simulink model "test_kat_adc_fab_inter"  (Simulink 7.2)
settings: Solver=ode45  StartTime=0.0  StopTime=10.0  RelTol=1e-3
libraries: xbsIndex_r4 x171, simulink x58, dspsigops x24, xps_library x5, casper_library_scopes x2
settings Model: Creator=dave  LastModifiedBy=root
settings OptimizationCC: InitFltsAndDblsToZero=on

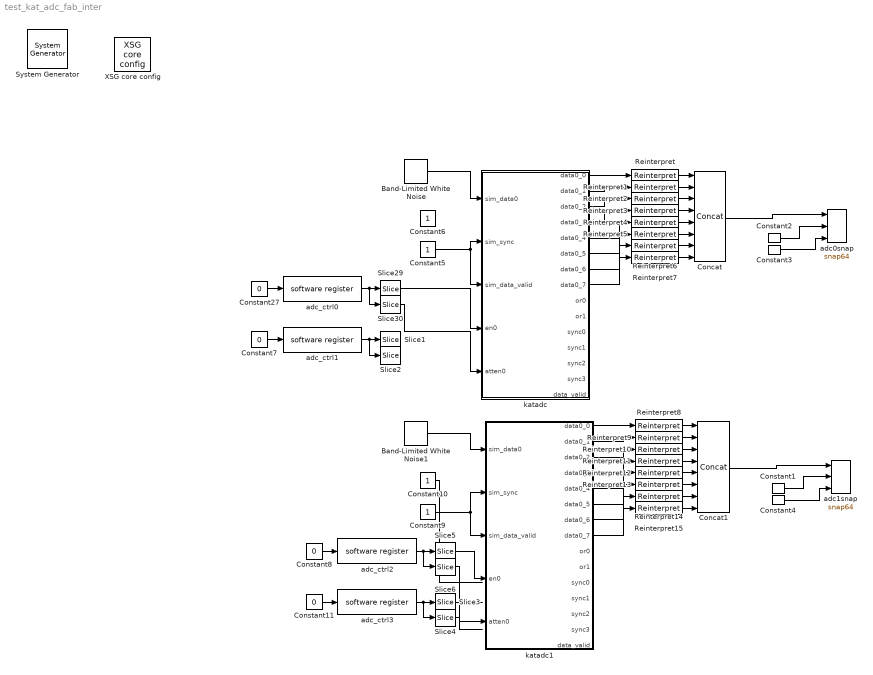
== system test_kat_adc_fab_inter ==
  " System Generator" : xbsIndex_r4/ System Generator  Tag=genX  SystemSampleTime=-1  xilinxfamily=virtex5  part=xc5vsx95t  speed=-1  package=ff1136  synthesis_tool=XST  clock_wrapper=Clock Enables  directory=./test_kat_adc_fab_inter/sysgen  testbench=off  simulink_period=1  sysclk_period=4  dcm_input_clock_period=100  incr_netlist=off  trim_vbits=Everywhere in SubSystem  dbl_ovrd=According to Block Masks  core_generation=According to Block Masks  run_coregen=off  deprecated_control=off  eval_field=0  block_type=sysgen
      settings: block_version=10.1.3
  Band-Limited White Noise : simulink/Sources/Band-Limited White Noise  SystemSampleTime=-1  Cov=[0.1]  Ts=0.25  seed=[23341]
  Band-Limited White Noise1 : simulink/Sources/Band-Limited White Noise  SystemSampleTime=-1  Cov=[0.1]  Ts=0.25  seed=[23341]
  Concat : xbsIndex_r4/Concat  num_inputs=8  dbl_ovrd=off  block_type=concat
      settings: block_version=11.3
  Concat1 : xbsIndex_r4/Concat  num_inputs=8  dbl_ovrd=off  block_type=concat
      settings: block_version=11.3
  Constant{1..4} (4 alike) : xbsIndex_r4/Constant  arith_type=Boolean  const=0  n_bits=16  bin_pt=14  explicit_period=on  period=1  equ=P=C  opselect=C  inp2=PCIN>>17  opr=+  inp1=P  carry=CIN  dbl_ovrd=off  block_type=constant
      settings: block_version=11.3
  Constant{5..6,9..10} (4 alike) : Constant  OutDataType=sfix(16)  OutScaling=2^0  SampleTime=1
  Constant{7..8,11,27} (4 alike) : Constant  Value=0  OutDataType=sfix(16)  OutScaling=2^0
  Reinterpret{,1..15} (16 alike) : xbsIndex_r4/Reinterpret  force_arith_type=on  arith_type=Unsigned  force_bin_pt=on  bin_pt=0  block_type=reinterpret
      settings: infoedit="Changes signal type without altering the binary representation.   You can changed the signal between signed and unsigned, and relocate the binary point.<br><br>Hardware notes: In hardware this block costs nothing.<br><br>Example:  Suppose the input is 6 bits wide, signed, with 2 fractional bits, and the output is forced to unsigned with 0 fractional bits.  Then an input of -2.0 (1110.00 in binary 2's complement) becomes an output of 56 (111000 in binary)."  block_version=11.3
  Slice{1,3,5,29} (4 alike) : xbsIndex_r4/Slice  nbits=1  boolean_output=on  mode=Upper Bit Location + Width  bit1=0  base1=MSB of Input  bit0=0  base0=LSB of Input  dbl_ovrd=off  block_type=slice
  Slice{2,4,6,30} (4 alike) : xbsIndex_r4/Slice  nbits=6  boolean_output=off  mode=Lower Bit Location + Width  bit1=0  base1=MSB of Input  bit0=0  base0=LSB of Input  dbl_ovrd=off  block_type=slice
  XSG core config : xps_library/XSG core config  Tag=xps:xsg  SystemSampleTime=-1  hw_sys=ROACH:sx95t  ibob_linux=off  clk_src=adc0_clk  iBOB_clk_src=sys_clk  BEE2_ctrl_clk_src=sys_clk  BEE2_usr_clk_src=sys_clk  ROACH_clk_src=adc0_clk  CORR_clk_src=sys_clk  gpio_clk_io_group=iBOB:sma  gpio_clk_bit_index=0  clk_rate=250  sample_period=1  synthesis_tool=XST  mpc_type=powerpc440_ext
  adc0snap : casper_library_scopes/snap64  SystemSampleTime=-1  nsamples=11
  adc1snap : casper_library_scopes/snap64  SystemSampleTime=-1  nsamples=11
  adc_ctrl0 : xps_library/software register  Tag=xps:sw_reg  SystemSampleTime=-1  io_dir=From Processor  arith_type=Unsigned  bitwidth=32  bin_pt=0  sample_period=1  gw_name=test_kat_adc_fab_inter_adc_ctrl0_user_data_out
      link override poco_cd_tr0_ld_time_msb_user_data_out: arith_type=Unsigned  n_bits=32  bin_pt=0  period=1
      link override poco_dram_vacc_r001_cd_tr0_ld_time_msb_user_data_out: arith_type=Unsigned  n_bits=32  bin_pt=0  period=1
      link override poco_dram_vacc_r002_cd_tr0_ld_time_msb_user_data_out: arith_type=Unsigned  n_bits=32  bin_pt=0  period=1
      link override poco_dram_vacc_r003_cd_tr0_ld_time_msb_user_data_out: arith_type=Unsigned  n_bits=32  bin_pt=0  period=1
      link override poco_dram_vacc_r004_cd_tr0_ld_time_msb_user_data_out: arith_type=Unsigned  n_bits=32  bin_pt=0  period=1
      link override poco_dram_vacc_r005_cd_tr0_ld_time_msb_user_data_out: arith_type=Unsigned  n_bits=32  bin_pt=0  period=1
      link override poco_dram_vacc_r006_cd_tr0_ld_time_msb_user_data_out: arith_type=Unsigned  n_bits=32  bin_pt=0  period=1
      link override poco_r006_cd_tr0_ld_time_msb_user_data_out: arith_type=Unsigned  n_bits=32  bin_pt=0  period=1
      link override poco_red_cd_ld_time_msb_user_data_out: arith_type=Unsigned  n_bits=32  bin_pt=0  period=1
      link override poco_ref_roach_adc0_cd_ld_time_msb_user_data_out: arith_type=Unsigned  n_bits=32  bin_pt=0  period=1
      link override poco_ref_roach_reduced_adc0_cd_ld_time_msb_user_data_out: arith_type=Unsigned  n_bits=32  bin_pt=0  period=1
      link override poco_roach_cd_tr0_ld_time_msb_user_data_out: arith_type=Unsigned  n_bits=32  bin_pt=0  period=1
      link override poco_roach_r006_cd_tr0_ld_time_msb_user_data_out: arith_type=Unsigned  n_bits=32  bin_pt=0  period=1
      link override poco_roach_r007_cd_tr0_ld_time_msb_user_data_out: arith_type=Unsigned  n_bits=32  bin_pt=0  period=1
      link override poco_roach_red_adc0_cd_ld_time_msb_user_data_out: arith_type=Unsigned  n_bits=32  bin_pt=0  period=1
      link override poco_roach_vacc_r006_cd_tr0_ld_time_msb_user_data_out: arith_type=Unsigned  n_bits=32  bin_pt=0  period=1
  adc_ctrl1 : xps_library/software register  Tag=xps:sw_reg  SystemSampleTime=-1  io_dir=From Processor  arith_type=Unsigned  bitwidth=32  bin_pt=0  sample_period=1  gw_name=test_kat_adc_fab_inter_adc_ctrl1_user_data_out
      link override poco_cd_tr0_ld_time_msb_user_data_out: arith_type=Unsigned  n_bits=32  bin_pt=0  period=1
      link override poco_dram_vacc_r001_cd_tr0_ld_time_msb_user_data_out: arith_type=Unsigned  n_bits=32  bin_pt=0  period=1
      link override poco_dram_vacc_r002_cd_tr0_ld_time_msb_user_data_out: arith_type=Unsigned  n_bits=32  bin_pt=0  period=1
      link override poco_dram_vacc_r003_cd_tr0_ld_time_msb_user_data_out: arith_type=Unsigned  n_bits=32  bin_pt=0  period=1
      link override poco_dram_vacc_r004_cd_tr0_ld_time_msb_user_data_out: arith_type=Unsigned  n_bits=32  bin_pt=0  period=1
      link override poco_dram_vacc_r005_cd_tr0_ld_time_msb_user_data_out: arith_type=Unsigned  n_bits=32  bin_pt=0  period=1
      link override poco_dram_vacc_r006_cd_tr0_ld_time_msb_user_data_out: arith_type=Unsigned  n_bits=32  bin_pt=0  period=1
      link override poco_r006_cd_tr0_ld_time_msb_user_data_out: arith_type=Unsigned  n_bits=32  bin_pt=0  period=1
      link override poco_red_cd_ld_time_msb_user_data_out: arith_type=Unsigned  n_bits=32  bin_pt=0  period=1
      link override poco_ref_roach_adc0_cd_ld_time_msb_user_data_out: arith_type=Unsigned  n_bits=32  bin_pt=0  period=1
      link override poco_ref_roach_reduced_adc0_cd_ld_time_msb_user_data_out: arith_type=Unsigned  n_bits=32  bin_pt=0  period=1
      link override poco_roach_cd_tr0_ld_time_msb_user_data_out: arith_type=Unsigned  n_bits=32  bin_pt=0  period=1
      link override poco_roach_r006_cd_tr0_ld_time_msb_user_data_out: arith_type=Unsigned  n_bits=32  bin_pt=0  period=1
      link override poco_roach_r007_cd_tr0_ld_time_msb_user_data_out: arith_type=Unsigned  n_bits=32  bin_pt=0  period=1
      link override poco_roach_red_adc0_cd_ld_time_msb_user_data_out: arith_type=Unsigned  n_bits=32  bin_pt=0  period=1
      link override poco_roach_vacc_r006_cd_tr0_ld_time_msb_user_data_out: arith_type=Unsigned  n_bits=32  bin_pt=0  period=1
  adc_ctrl2 : xps_library/software register  Tag=xps:sw_reg  SystemSampleTime=-1  io_dir=From Processor  arith_type=Unsigned  bitwidth=32  bin_pt=0  sample_period=1  gw_name=test_kat_adc_fab_inter_adc_ctrl2_user_data_out
      link override poco_cd_tr0_ld_time_msb_user_data_out: arith_type=Unsigned  n_bits=32  bin_pt=0  period=1
      link override poco_dram_vacc_r001_cd_tr0_ld_time_msb_user_data_out: arith_type=Unsigned  n_bits=32  bin_pt=0  period=1
      link override poco_dram_vacc_r002_cd_tr0_ld_time_msb_user_data_out: arith_type=Unsigned  n_bits=32  bin_pt=0  period=1
      link override poco_dram_vacc_r003_cd_tr0_ld_time_msb_user_data_out: arith_type=Unsigned  n_bits=32  bin_pt=0  period=1
      link override poco_dram_vacc_r004_cd_tr0_ld_time_msb_user_data_out: arith_type=Unsigned  n_bits=32  bin_pt=0  period=1
      link override poco_dram_vacc_r005_cd_tr0_ld_time_msb_user_data_out: arith_type=Unsigned  n_bits=32  bin_pt=0  period=1
      link override poco_dram_vacc_r006_cd_tr0_ld_time_msb_user_data_out: arith_type=Unsigned  n_bits=32  bin_pt=0  period=1
      link override poco_r006_cd_tr0_ld_time_msb_user_data_out: arith_type=Unsigned  n_bits=32  bin_pt=0  period=1
      link override poco_red_cd_ld_time_msb_user_data_out: arith_type=Unsigned  n_bits=32  bin_pt=0  period=1
      link override poco_ref_roach_adc0_cd_ld_time_msb_user_data_out: arith_type=Unsigned  n_bits=32  bin_pt=0  period=1
      link override poco_ref_roach_reduced_adc0_cd_ld_time_msb_user_data_out: arith_type=Unsigned  n_bits=32  bin_pt=0  period=1
      link override poco_roach_cd_tr0_ld_time_msb_user_data_out: arith_type=Unsigned  n_bits=32  bin_pt=0  period=1
      link override poco_roach_r006_cd_tr0_ld_time_msb_user_data_out: arith_type=Unsigned  n_bits=32  bin_pt=0  period=1
      link override poco_roach_r007_cd_tr0_ld_time_msb_user_data_out: arith_type=Unsigned  n_bits=32  bin_pt=0  period=1
      link override poco_roach_red_adc0_cd_ld_time_msb_user_data_out: arith_type=Unsigned  n_bits=32  bin_pt=0  period=1
      link override poco_roach_vacc_r006_cd_tr0_ld_time_msb_user_data_out: arith_type=Unsigned  n_bits=32  bin_pt=0  period=1
  adc_ctrl3 : xps_library/software register  Tag=xps:sw_reg  SystemSampleTime=-1  io_dir=From Processor  arith_type=Unsigned  bitwidth=32  bin_pt=0  sample_period=1  gw_name=test_kat_adc_fab_inter_adc_ctrl3_user_data_out
      link override poco_cd_tr0_ld_time_msb_user_data_out: arith_type=Unsigned  n_bits=32  bin_pt=0  period=1
      link override poco_dram_vacc_r001_cd_tr0_ld_time_msb_user_data_out: arith_type=Unsigned  n_bits=32  bin_pt=0  period=1
      link override poco_dram_vacc_r002_cd_tr0_ld_time_msb_user_data_out: arith_type=Unsigned  n_bits=32  bin_pt=0  period=1
      link override poco_dram_vacc_r003_cd_tr0_ld_time_msb_user_data_out: arith_type=Unsigned  n_bits=32  bin_pt=0  period=1
      link override poco_dram_vacc_r004_cd_tr0_ld_time_msb_user_data_out: arith_type=Unsigned  n_bits=32  bin_pt=0  period=1
      link override poco_dram_vacc_r005_cd_tr0_ld_time_msb_user_data_out: arith_type=Unsigned  n_bits=32  bin_pt=0  period=1
      link override poco_dram_vacc_r006_cd_tr0_ld_time_msb_user_data_out: arith_type=Unsigned  n_bits=32  bin_pt=0  period=1
      link override poco_r006_cd_tr0_ld_time_msb_user_data_out: arith_type=Unsigned  n_bits=32  bin_pt=0  period=1
      link override poco_red_cd_ld_time_msb_user_data_out: arith_type=Unsigned  n_bits=32  bin_pt=0  period=1
      link override poco_ref_roach_adc0_cd_ld_time_msb_user_data_out: arith_type=Unsigned  n_bits=32  bin_pt=0  period=1
      link override poco_ref_roach_reduced_adc0_cd_ld_time_msb_user_data_out: arith_type=Unsigned  n_bits=32  bin_pt=0  period=1
      link override poco_roach_cd_tr0_ld_time_msb_user_data_out: arith_type=Unsigned  n_bits=32  bin_pt=0  period=1
      link override poco_roach_r006_cd_tr0_ld_time_msb_user_data_out: arith_type=Unsigned  n_bits=32  bin_pt=0  period=1
      link override poco_roach_r007_cd_tr0_ld_time_msb_user_data_out: arith_type=Unsigned  n_bits=32  bin_pt=0  period=1
      link override poco_roach_red_adc0_cd_ld_time_msb_user_data_out: arith_type=Unsigned  n_bits=32  bin_pt=0  period=1
      link override poco_roach_vacc_r006_cd_tr0_ld_time_msb_user_data_out: arith_type=Unsigned  n_bits=32  bin_pt=0  period=1
  katadc : Subsystem  Tag=xps:katadc  AncestorBlock=xps_library/katadc  mask(katadc){adc_brd=adc0, adc_interleave=on, bypass_auto=off, en_gain=on, adc_clk_rate=900, sample_period=1}
      mask prompts: adc_brd "ADC board"; adc_interleave "ADC interleave mode"; bypass_auto "Bypass auto config"; en_gain "Enable gain"; adc_clk_rate "ADC sampling rate (MHz)"; sample_period "Sample period"
      mask init:
      | name = gcb;
      | katadc_init(gcb, ...
      |     'name', name, ...
      |     'adc_brd', adc_brd, ...
      |     'adc_interleave', adc_interleave, ...
      |     'bypass_auto', bypass_auto, ...
      |     'en_gain', en_gain, ...
      |     'adc_clk_rate', adc_clk_rate, ...
      |     'sample_period', sample_period);
      mask StyleString: popup(adc0|adc1),checkbox,checkbox,checkbox,edit,edit
  katadc1 : Subsystem  Tag=xps:katadc  AncestorBlock=xps_library/katadc  mask(katadc){adc_brd=adc1, adc_interleave=on, bypass_auto=on, en_gain=on, adc_clk_rate=900, sample_period=1}
      mask prompts: adc_brd "ADC board"; adc_interleave "ADC interleave mode"; bypass_auto "Bypass auto config"; en_gain "Enable gain"; adc_clk_rate "ADC sampling rate (MHz)"; sample_period "Sample period"
      mask init: same as test_kat_adc_fab_inter/katadc
      mask StyleString: popup(adc0|adc1),checkbox,checkbox,checkbox,edit,edit
  wires:
  Reinterpret/1 -> Concat/1
  Reinterpret1/1 -> Concat/2
  Reinterpret2/1 -> Concat/3
  Reinterpret3/1 -> Concat/4
  Reinterpret4/1 -> Concat/5
  Reinterpret5/1 -> Concat/6
  Reinterpret6/1 -> Concat/7
  Reinterpret7/1 -> Concat/8
  Concat/1 -> adc0snap/1
  Constant2/1 -> adc0snap/2
  Constant3/1 -> adc0snap/3
  Reinterpret8/1 -> Concat1/1
  Reinterpret9/1 -> Concat1/2
  Reinterpret10/1 -> Concat1/3
  Reinterpret11/1 -> Concat1/4
  Reinterpret12/1 -> Concat1/5
  Reinterpret13/1 -> Concat1/6
  Reinterpret14/1 -> Concat1/7
  Reinterpret15/1 -> Concat1/8
  Concat1/1 -> adc1snap/1
  Constant1/1 -> adc1snap/2
  Constant4/1 -> adc1snap/3
  Constant5/1 -> katadc/2(sim_sync), katadc/3(sim_data_valid)
  Band-Limited White Noise/1 -> katadc/1(sim_data0)
  Constant27/1 -> adc_ctrl0/1
  adc_ctrl0/1 -> Slice29/1, Slice30/1
  Slice29/1 -> katadc/4(en0)
  Slice30/1 -> katadc/5(atten0)
  Constant7/1 -> adc_ctrl1/1
  adc_ctrl1/1 -> Slice2/1, Slice1/1
  Constant9/1 -> katadc1/2(sim_sync), katadc1/3(sim_data_valid)
  Constant10/1 -> ?
  Band-Limited White Noise1/1 -> katadc1/1(sim_data0)
  Constant8/1 -> adc_ctrl2/1
  adc_ctrl2/1 -> Slice5/1, Slice6/1
  Slice5/1 -> katadc1/4(en0)
  Slice6/1 -> katadc1/5(atten0)
  Constant11/1 -> adc_ctrl3/1
  adc_ctrl3/1 -> Slice4/1, Slice3/1
  Slice3/1 -> ?
  Slice4/1 -> ?
  katadc/1(data0_0) -> Reinterpret/1
  katadc/2(data0_1) -> Reinterpret1/1
  katadc/3(data0_2) -> Reinterpret2/1
  katadc/4(data0_3) -> Reinterpret3/1
  katadc/5(data0_4) -> Reinterpret4/1
  katadc/6(data0_5) -> Reinterpret5/1
  katadc/7(data0_6) -> Reinterpret6/1
  katadc/8(data0_7) -> Reinterpret7/1
  katadc1/1(data0_0) -> Reinterpret8/1
  katadc1/2(data0_1) -> Reinterpret9/1
  katadc1/3(data0_2) -> Reinterpret10/1
  katadc1/4(data0_3) -> Reinterpret11/1
  katadc1/5(data0_4) -> Reinterpret12/1
  katadc1/6(data0_5) -> Reinterpret13/1
  katadc1/7(data0_6) -> Reinterpret14/1
  katadc1/8(data0_7) -> Reinterpret15/1

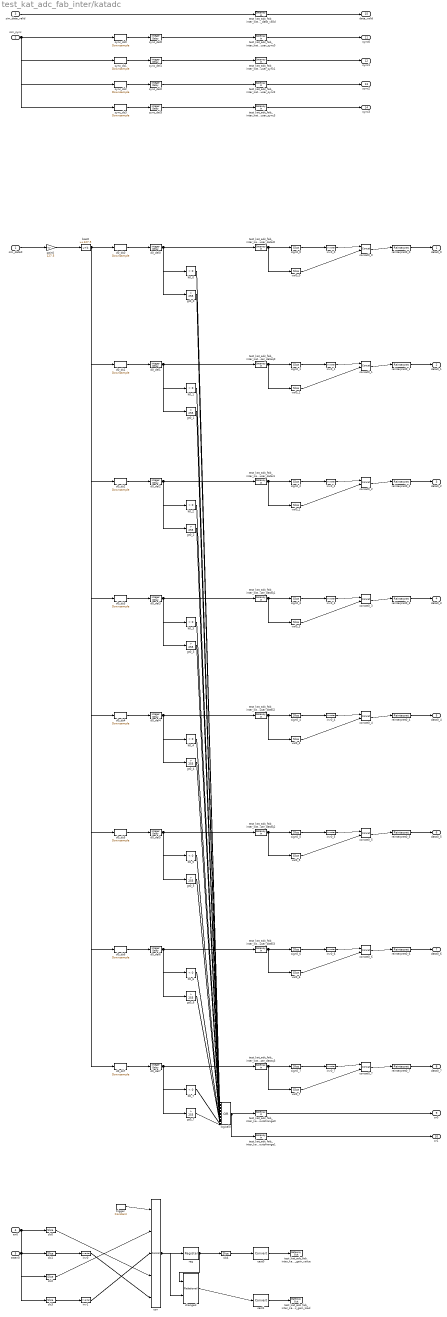
== system test_kat_adc_fab_inter/katadc ==
  sim_data0 : Inport
  sim_sync : Inport  Port=2
  sim_data_valid : Inport  Port=3
  en0 : Inport  Port=4
  atten0 : Inport  Port=5
  bias0 : Bias  Bias=127.5  SaturateOnIntegerOverflow=on
  cast0 : xbsIndex_r4/Convert  arith_type=Unsigned  n_bits=14  bin_pt=0  quantization=Truncate  overflow=Wrap  latency=0  dbl_ovrd=off  pipeline=off  block_type=convert
      settings: block_version=11.4
  cast1 : xbsIndex_r4/Convert  arith_type=Boolean  n_bits=16  bin_pt=14  quantization=Truncate  overflow=Wrap  latency=0  dbl_ovrd=off  pipeline=off  block_type=convert
      settings: block_version=11.4
  changed : xbsIndex_r4/Relational  mode=a!=b  en=off  latency=1  dbl_ovrd=off  block_type=relational
  con : xbsIndex_r4/Concat  num_inputs=5  dbl_ovrd=off  block_type=concat
  concat0_{0..7} (8 alike) : xbsIndex_r4/Concat  num_inputs=2  dbl_ovrd=off  block_type=concat
  d0_del0 : simulink/Discrete/Integer Delay  vinit=0.0  samptime=-1  NumDelays=2
  d0_del{1..7} (7 alike) : simulink/Discrete/Integer Delay  vinit=0.0  samptime=-1  NumDelays=1
  d0_ds0 : dspsigops/Downsample  N=8  phase=0  ic=0  smode=Allow multirate  fmode=Maintain input frame size
  d0_ds1 : dspsigops/Downsample  N=8  phase=1  ic=0  smode=Allow multirate  fmode=Maintain input frame size
  d0_ds2 : dspsigops/Downsample  N=8  phase=2  ic=0  smode=Allow multirate  fmode=Maintain input frame size
  d0_ds3 : dspsigops/Downsample  N=8  phase=3  ic=0  smode=Allow multirate  fmode=Maintain input frame size
  d0_ds4 : dspsigops/Downsample  N=8  phase=4  ic=0  smode=Allow multirate  fmode=Maintain input frame size
  d0_ds5 : dspsigops/Downsample  N=8  phase=5  ic=0  smode=Allow multirate  fmode=Maintain input frame size
  d0_ds6 : dspsigops/Downsample  N=8  phase=6  ic=0  smode=Allow multirate  fmode=Maintain input frame size
  d0_ds7 : dspsigops/Downsample  N=8  phase=7  ic=0  smode=Allow multirate  fmode=Maintain input frame size
  gain0 : Gain  Gain=127.5  SaturateOnIntegerOverflow=on  OutDataTypeStr=Inherit: Same as input  ParamDataTypeStr=Inherit: Same as input
  gt0_{0..7} (8 alike) : simulink/Logic and Bit Operations/Compare To Constant  SystemSampleTime=-1  relop=>  const=255  LogicOutDataTypeMode=boolean  ZeroCross=off
  inv0 : xbsIndex_r4/Inverter  en=off  latency=0  dbl_ovrd=off  block_type=inv
      settings: block_version=11.4
  inv0_{0..7} (8 alike) : xbsIndex_r4/Inverter  en=off  latency=0  dbl_ovrd=off  block_type=inv
      settings: block_version=11.4
  inv1 : xbsIndex_r4/Inverter  en=off  latency=0  dbl_ovrd=off  block_type=inv
      settings: block_version=11.4
  logical0 : Logic  Operator=OR  Inputs=16  AllPortsSameDT=off  OutDataTypeMode=boolean  OutDataTypeStr=boolean
  lt0_{0..7} (8 alike) : simulink/Logic and Bit Operations/Compare To Constant  SystemSampleTime=-1  relop=<  const=0  LogicOutDataTypeMode=boolean  ZeroCross=off
  reg : xbsIndex_r4/Register  init=0  rst=off  en=off  dbl_ovrd=off  block_type=register
      settings: block_version=11.4
  reinterpret0_{0..7} (8 alike) : xbsIndex_r4/Reinterpret  force_arith_type=on  arith_type="Signed  (2's comp)"  force_bin_pt=on  bin_pt=7  block_type=reinterpret
      settings: infoedit="Changes signal type without altering the binary representation.   You can changed the signal between signed and unsigned, and relocate the binary point.<br><br>Hardware notes: In hardware this block costs nothing.<br><br>Example:  Suppose the input is 6 bits wide, signed, with 2 fractional bits, and the output is forced to unsigned with 0 fractional bits.  Then an input of -2.0 (1110.00 in binary 2's complement) becomes an output of 56 (111000 in binary)."
  sign0_{0..7} (8 alike) : xbsIndex_r4/Slice  nbits=1  boolean_output=off  mode=Upper Bit Location + Width  bit1=0  base1=MSB of Input  bit0=0  base0=MSB of Input  dbl_ovrd=off  block_type=slice
  slc0 : xbsIndex_r4/Slice  nbits=1  boolean_output=off  mode=Lower Bit Location + Width  bit1=0  base1=MSB of Input  bit0=0  base0=LSB of Input  dbl_ovrd=off  block_type=slice
  slc1 : xbsIndex_r4/Slice  nbits=6  boolean_output=off  mode=Lower Bit Location + Width  bit1=0  base1=MSB of Input  bit0=0  base0=LSB of Input  dbl_ovrd=off  block_type=slice
  slc2 : xbsIndex_r4/Slice  nbits=1  boolean_output=off  mode=Lower Bit Location + Width  bit1=0  base1=MSB of Input  bit0=0  base0=LSB of Input  dbl_ovrd=off  block_type=slice
  slc3 : xbsIndex_r4/Slice  nbits=6  boolean_output=off  mode=Lower Bit Location + Width  bit1=0  base1=MSB of Input  bit0=0  base0=LSB of Input  dbl_ovrd=off  block_type=slice
  slc4 : xbsIndex_r4/Slice  nbits=14  boolean_output=off  mode=Lower Bit Location + Width  bit1=0  base1=MSB of Input  bit0=0  base0=LSB of Input  dbl_ovrd=off  block_type=slice
  sync_del0 : simulink/Discrete/Integer Delay  vinit=0.0  samptime=-1  NumDelays=2
  sync_del1 : simulink/Discrete/Integer Delay  vinit=0.0  samptime=-1  NumDelays=1
  sync_del2 : simulink/Discrete/Integer Delay  vinit=0.0  samptime=-1  NumDelays=1
  sync_del3 : simulink/Discrete/Integer Delay  vinit=0.0  samptime=-1  NumDelays=1
  sync_ds0 : dspsigops/Downsample  N=8  phase=0  ic=0  smode=Allow multirate  fmode=Maintain input frame size
  sync_ds1 : dspsigops/Downsample  N=8  phase=2  ic=0  smode=Allow multirate  fmode=Maintain input frame size
  sync_ds2 : dspsigops/Downsample  N=8  phase=4  ic=0  smode=Allow multirate  fmode=Maintain input frame size
  sync_ds3 : dspsigops/Downsample  N=8  phase=6  ic=0  smode=Allow multirate  fmode=Maintain input frame size
  test_kat_adc_fab_inter_katadc_gain_load : xbsIndex_r4/Gateway Out  hdl_port=on  timing_constraint=None  locs_specified=off  LOCs={}  block_type=gatewayout
      settings: infoedit="Gateway out block.  Converts Xilinx fixed point inputs into ouputs of type Simulink integer, double, or fixed point.<br><br>Hardware notes:  In hardware these blocks become top level output ports or are discarded, depending on how they are configured."  block_version=11.4
  test_kat_adc_fab_inter_katadc_gain_value : xbsIndex_r4/Gateway Out  hdl_port=on  timing_constraint=None  locs_specified=off  LOCs={}  block_type=gatewayout
      settings: infoedit="Gateway out block.  Converts Xilinx fixed point inputs into ouputs of type Simulink integer, double, or fixed point.<br><br>Hardware notes:  In hardware these blocks become top level output ports or are discarded, depending on how they are configured."  block_version=11.4
  test_kat_adc_fab_inter_katadc_user_data_valid : xbsIndex_r4/Gateway In  arith_type=Boolean  n_bits=16  bin_pt=14  quantization="Round  (unbiased: +/- Inf)"  overflow=Saturate  period=1  dbl_ovrd=off  timing_constraint=None  locs_specified=off  LOCs={}  hdl_port=on  block_type=gatewayin
      settings: infoedit="Gateway in block.  Converts inputs of type Simulink integer, double and fixed point to  Xilinx fixed point type.<br><br>Hardware notes:  In hardware these blocks become top level input ports."  block_version=11.4
  test_kat_adc_fab_inter_katadc_user_datai{0..3} (4 alike) : xbsIndex_r4/Gateway In  arith_type="Signed  (2's comp)"  n_bits=8  bin_pt=0  quantization="Round  (unbiased: +/- Inf)"  overflow=Saturate  period=1  dbl_ovrd=off  timing_constraint=None  locs_specified=off  LOCs={}  hdl_port=on  block_type=gatewayin
      settings: infoedit="Gateway in block.  Converts inputs of type Simulink integer, double and fixed point to  Xilinx fixed point type.<br><br>Hardware notes:  In hardware these blocks become top level input ports."  block_version=11.4
  test_kat_adc_fab_inter_katadc_user_dataq{0..3} (4 alike) : xbsIndex_r4/Gateway In  arith_type="Signed  (2's comp)"  n_bits=8  bin_pt=0  quantization="Round  (unbiased: +/- Inf)"  overflow=Saturate  period=1  dbl_ovrd=off  timing_constraint=None  locs_specified=off  LOCs={}  hdl_port=on  block_type=gatewayin
      settings: infoedit="Gateway in block.  Converts inputs of type Simulink integer, double and fixed point to  Xilinx fixed point type.<br><br>Hardware notes:  In hardware these blocks become top level input ports."  block_version=11.4
  test_kat_adc_fab_inter_katadc_user_outofrange0 : xbsIndex_r4/Gateway In  arith_type=Boolean  n_bits=16  bin_pt=14  quantization="Round  (unbiased: +/- Inf)"  overflow=Saturate  period=1  dbl_ovrd=off  timing_constraint=None  locs_specified=off  LOCs={}  hdl_port=on  block_type=gatewayin
      settings: infoedit="Gateway in block.  Converts inputs of type Simulink integer, double and fixed point to  Xilinx fixed point type.<br><br>Hardware notes:  In hardware these blocks become top level input ports."  block_version=11.4
  test_kat_adc_fab_inter_katadc_user_outofrange1 : xbsIndex_r4/Gateway In  arith_type=Boolean  n_bits=16  bin_pt=14  quantization="Round  (unbiased: +/- Inf)"  overflow=Saturate  period=1  dbl_ovrd=off  timing_constraint=None  locs_specified=off  LOCs={}  hdl_port=on  block_type=gatewayin
      settings: infoedit="Gateway in block.  Converts inputs of type Simulink integer, double and fixed point to  Xilinx fixed point type.<br><br>Hardware notes:  In hardware these blocks become top level input ports."  block_version=11.4
  test_kat_adc_fab_inter_katadc_user_sync{0..3} (4 alike) : xbsIndex_r4/Gateway In  arith_type=Boolean  n_bits=16  bin_pt=14  quantization="Round  (unbiased: +/- Inf)"  overflow=Saturate  period=1  dbl_ovrd=off  timing_constraint=None  locs_specified=off  LOCs={}  hdl_port=on  block_type=gatewayin
      settings: infoedit="Gateway in block.  Converts inputs of type Simulink integer, double and fixed point to  Xilinx fixed point type.<br><br>Hardware notes:  In hardware these blocks become top level input ports."  block_version=11.4
  trigger : xbsIndex_r4/Constant  arith_type=Unsigned  const=1  n_bits=1  bin_pt=0  explicit_period=off  period=1  equ=P=C  opselect=C  inp2=PCIN>>17  opr=+  inp1=P  carry=CIN  dbl_ovrd=off  block_type=constant
      settings: block_version=11.4
  val0_{0..7} (8 alike) : xbsIndex_r4/Slice  nbits=7  boolean_output=off  mode=Lower Bit Location + Width  bit1=0  base1=LSB of Input  bit0=0  base0=LSB of Input  dbl_ovrd=off  block_type=slice
  data0_0 : Outport
  data0_1 : Outport  Port=2
  data0_2 : Outport  Port=3
  data0_3 : Outport  Port=4
  data0_4 : Outport  Port=5
  data0_5 : Outport  Port=6
  data0_6 : Outport  Port=7
  data0_7 : Outport  Port=8
  or0 : Outport  Port=9
  or1 : Outport  Port=10
  sync0 : Outport  Port=11
  sync1 : Outport  Port=12
  sync2 : Outport  Port=13
  sync3 : Outport  Port=14
  data_valid : Outport  Port=15
  wires:
  sim_data0/1 -> gain0/1
  gain0/1 -> bias0/1
  bias0/1 -> d0_ds0/1, d0_ds1/1, d0_ds2/1, d0_ds3/1, d0_ds4/1, d0_ds5/1, d0_ds6/1, d0_ds7/1
  d0_ds0/1 -> d0_del0/1
  d0_del0/1 -> test_kat_adc_fab_inter_katadc_user_datai0/1, lt0_0/1, gt0_0/1
  test_kat_adc_fab_inter_katadc_user_datai0/1 -> sign0_0/1, val0_0/1
  sign0_0/1 -> inv0_0/1
  inv0_0/1 -> concat0_0/1
  val0_0/1 -> concat0_0/2
  concat0_0/1 -> reinterpret0_0/1
  reinterpret0_0/1 -> data0_0/1
  d0_ds1/1 -> d0_del1/1
  d0_del1/1 -> test_kat_adc_fab_inter_katadc_user_dataq0/1, lt0_1/1, gt0_1/1
  test_kat_adc_fab_inter_katadc_user_dataq0/1 -> sign0_1/1, val0_1/1
  sign0_1/1 -> inv0_1/1
  inv0_1/1 -> concat0_1/1
  val0_1/1 -> concat0_1/2
  concat0_1/1 -> reinterpret0_1/1
  reinterpret0_1/1 -> data0_1/1
  d0_ds2/1 -> d0_del2/1
  d0_del2/1 -> test_kat_adc_fab_inter_katadc_user_datai1/1, lt0_2/1, gt0_2/1
  test_kat_adc_fab_inter_katadc_user_datai1/1 -> sign0_2/1, val0_2/1
  sign0_2/1 -> inv0_2/1
  inv0_2/1 -> concat0_2/1
  val0_2/1 -> concat0_2/2
  concat0_2/1 -> reinterpret0_2/1
  reinterpret0_2/1 -> data0_2/1
  d0_ds3/1 -> d0_del3/1
  d0_del3/1 -> test_kat_adc_fab_inter_katadc_user_dataq1/1, lt0_3/1, gt0_3/1
  test_kat_adc_fab_inter_katadc_user_dataq1/1 -> sign0_3/1, val0_3/1
  sign0_3/1 -> inv0_3/1
  inv0_3/1 -> concat0_3/1
  val0_3/1 -> concat0_3/2
  concat0_3/1 -> reinterpret0_3/1
  reinterpret0_3/1 -> data0_3/1
  d0_ds4/1 -> d0_del4/1
  d0_del4/1 -> test_kat_adc_fab_inter_katadc_user_datai2/1, lt0_4/1, gt0_4/1
  test_kat_adc_fab_inter_katadc_user_datai2/1 -> sign0_4/1, val0_4/1
  sign0_4/1 -> inv0_4/1
  inv0_4/1 -> concat0_4/1
  val0_4/1 -> concat0_4/2
  concat0_4/1 -> reinterpret0_4/1
  reinterpret0_4/1 -> data0_4/1
  d0_ds5/1 -> d0_del5/1
  d0_del5/1 -> test_kat_adc_fab_inter_katadc_user_dataq2/1, lt0_5/1, gt0_5/1
  test_kat_adc_fab_inter_katadc_user_dataq2/1 -> sign0_5/1, val0_5/1
  sign0_5/1 -> inv0_5/1
  inv0_5/1 -> concat0_5/1
  val0_5/1 -> concat0_5/2
  concat0_5/1 -> reinterpret0_5/1
  reinterpret0_5/1 -> data0_5/1
  d0_ds6/1 -> d0_del6/1
  d0_del6/1 -> test_kat_adc_fab_inter_katadc_user_datai3/1, lt0_6/1, gt0_6/1
  test_kat_adc_fab_inter_katadc_user_datai3/1 -> sign0_6/1, val0_6/1
  sign0_6/1 -> inv0_6/1
  inv0_6/1 -> concat0_6/1
  val0_6/1 -> concat0_6/2
  concat0_6/1 -> reinterpret0_6/1
  reinterpret0_6/1 -> data0_6/1
  d0_ds7/1 -> d0_del7/1
  d0_del7/1 -> test_kat_adc_fab_inter_katadc_user_dataq3/1, lt0_7/1, gt0_7/1
  test_kat_adc_fab_inter_katadc_user_dataq3/1 -> sign0_7/1, val0_7/1
  sign0_7/1 -> inv0_7/1
  inv0_7/1 -> concat0_7/1
  val0_7/1 -> concat0_7/2
  concat0_7/1 -> reinterpret0_7/1
  reinterpret0_7/1 -> data0_7/1
  lt0_0/1 -> logical0/1
  gt0_0/1 -> logical0/2
  lt0_1/1 -> logical0/3
  gt0_1/1 -> logical0/4
  lt0_2/1 -> logical0/5
  gt0_2/1 -> logical0/6
  lt0_3/1 -> logical0/7
  gt0_3/1 -> logical0/8
  lt0_4/1 -> logical0/9
  gt0_4/1 -> logical0/10
  lt0_5/1 -> logical0/11
  gt0_5/1 -> logical0/12
  lt0_6/1 -> logical0/13
  gt0_6/1 -> logical0/14
  lt0_7/1 -> logical0/15
  gt0_7/1 -> logical0/16
  logical0/1 -> test_kat_adc_fab_inter_katadc_user_outofrange0/1, test_kat_adc_fab_inter_katadc_user_outofrange1/1
  test_kat_adc_fab_inter_katadc_user_outofrange0/1 -> or0/1
  test_kat_adc_fab_inter_katadc_user_outofrange1/1 -> or1/1
  sim_sync/1 -> sync_ds0/1, sync_ds1/1, sync_ds2/1, sync_ds3/1
  sync_ds0/1 -> sync_del0/1
  sync_del0/1 -> test_kat_adc_fab_inter_katadc_user_sync0/1
  test_kat_adc_fab_inter_katadc_user_sync0/1 -> sync0/1
  sync_ds1/1 -> sync_del1/1
  sync_del1/1 -> test_kat_adc_fab_inter_katadc_user_sync1/1
  test_kat_adc_fab_inter_katadc_user_sync1/1 -> sync1/1
  sync_ds2/1 -> sync_del2/1
  sync_del2/1 -> test_kat_adc_fab_inter_katadc_user_sync2/1
  test_kat_adc_fab_inter_katadc_user_sync2/1 -> sync2/1
  sync_ds3/1 -> sync_del3/1
  sync_del3/1 -> test_kat_adc_fab_inter_katadc_user_sync3/1
  test_kat_adc_fab_inter_katadc_user_sync3/1 -> sync3/1
  sim_data_valid/1 -> test_kat_adc_fab_inter_katadc_user_data_valid/1
  test_kat_adc_fab_inter_katadc_user_data_valid/1 -> data_valid/1
  en0/1 -> slc0/1, slc2/1
  atten0/1 -> slc1/1, slc3/1
  slc1/1 -> inv0/1
  slc3/1 -> inv1/1
  trigger/1 -> con/1
  slc0/1 -> con/4
  inv0/1 -> con/5
  slc2/1 -> con/2
  inv1/1 -> con/3
  con/1 -> reg/1, changed/2
  reg/1 -> changed/1, slc4/1
  slc4/1 -> cast0/1
  cast0/1 -> test_kat_adc_fab_inter_katadc_gain_value/1
  changed/1 -> cast1/1
  cast1/1 -> test_kat_adc_fab_inter_katadc_gain_load/1

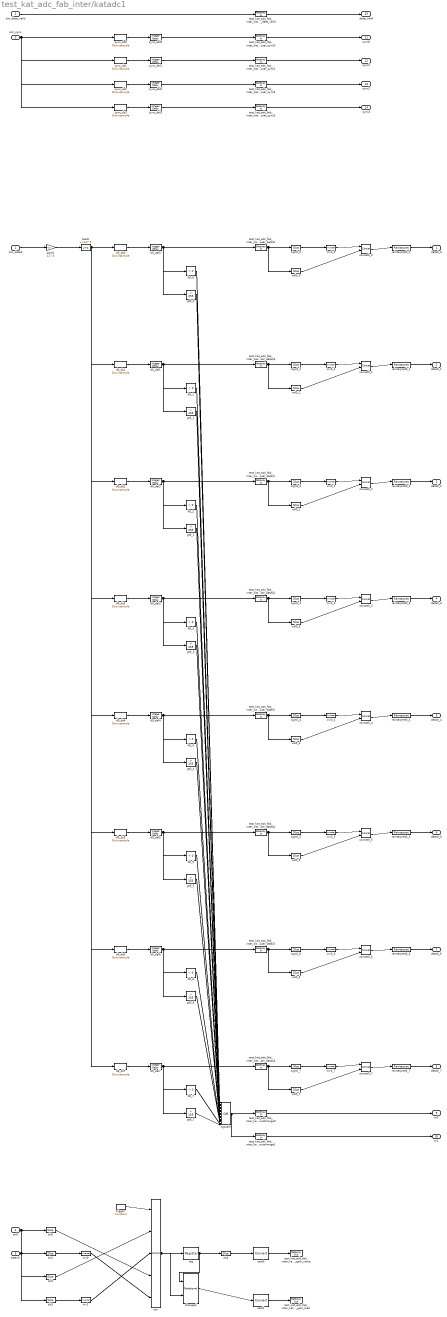
== system test_kat_adc_fab_inter/katadc1 ==
  sim_data0 : Inport
  sim_sync : Inport  Port=2
  sim_data_valid : Inport  Port=3
  en0 : Inport  Port=4
  atten0 : Inport  Port=5
  bias0 : Bias  Bias=127.5  SaturateOnIntegerOverflow=on
  cast0 : xbsIndex_r4/Convert  arith_type=Unsigned  n_bits=14  bin_pt=0  quantization=Truncate  overflow=Wrap  latency=0  dbl_ovrd=off  pipeline=off  block_type=convert
      settings: block_version=11.4
  cast1 : xbsIndex_r4/Convert  arith_type=Boolean  n_bits=16  bin_pt=14  quantization=Truncate  overflow=Wrap  latency=0  dbl_ovrd=off  pipeline=off  block_type=convert
      settings: block_version=11.4
  changed : xbsIndex_r4/Relational  mode=a!=b  en=off  latency=1  dbl_ovrd=off  block_type=relational
  con : xbsIndex_r4/Concat  num_inputs=5  dbl_ovrd=off  block_type=concat
  concat0_{0..7} (8 alike) : xbsIndex_r4/Concat  num_inputs=2  dbl_ovrd=off  block_type=concat
  d0_del0 : simulink/Discrete/Integer Delay  vinit=0.0  samptime=-1  NumDelays=2
  d0_del{1..7} (7 alike) : simulink/Discrete/Integer Delay  vinit=0.0  samptime=-1  NumDelays=1
  d0_ds0 : dspsigops/Downsample  N=8  phase=0  ic=0  smode=Allow multirate  fmode=Maintain input frame size
  d0_ds1 : dspsigops/Downsample  N=8  phase=1  ic=0  smode=Allow multirate  fmode=Maintain input frame size
  d0_ds2 : dspsigops/Downsample  N=8  phase=2  ic=0  smode=Allow multirate  fmode=Maintain input frame size
  d0_ds3 : dspsigops/Downsample  N=8  phase=3  ic=0  smode=Allow multirate  fmode=Maintain input frame size
  d0_ds4 : dspsigops/Downsample  N=8  phase=4  ic=0  smode=Allow multirate  fmode=Maintain input frame size
  d0_ds5 : dspsigops/Downsample  N=8  phase=5  ic=0  smode=Allow multirate  fmode=Maintain input frame size
  d0_ds6 : dspsigops/Downsample  N=8  phase=6  ic=0  smode=Allow multirate  fmode=Maintain input frame size
  d0_ds7 : dspsigops/Downsample  N=8  phase=7  ic=0  smode=Allow multirate  fmode=Maintain input frame size
  gain0 : Gain  Gain=127.5  SaturateOnIntegerOverflow=on  OutDataTypeStr=Inherit: Same as input  ParamDataTypeStr=Inherit: Same as input
  gt0_{0..7} (8 alike) : simulink/Logic and Bit Operations/Compare To Constant  SystemSampleTime=-1  relop=>  const=255  LogicOutDataTypeMode=boolean  ZeroCross=off
  inv0 : xbsIndex_r4/Inverter  en=off  latency=0  dbl_ovrd=off  block_type=inv
      settings: block_version=11.4
  inv0_{0..7} (8 alike) : xbsIndex_r4/Inverter  en=off  latency=0  dbl_ovrd=off  block_type=inv
      settings: block_version=11.4
  inv1 : xbsIndex_r4/Inverter  en=off  latency=0  dbl_ovrd=off  block_type=inv
      settings: block_version=11.4
  logical0 : Logic  Operator=OR  Inputs=16  AllPortsSameDT=off  OutDataTypeMode=boolean  OutDataTypeStr=boolean
  lt0_{0..7} (8 alike) : simulink/Logic and Bit Operations/Compare To Constant  SystemSampleTime=-1  relop=<  const=0  LogicOutDataTypeMode=boolean  ZeroCross=off
  reg : xbsIndex_r4/Register  init=0  rst=off  en=off  dbl_ovrd=off  block_type=register
      settings: block_version=11.4
  reinterpret0_{0..7} (8 alike) : xbsIndex_r4/Reinterpret  force_arith_type=on  arith_type="Signed  (2's comp)"  force_bin_pt=on  bin_pt=7  block_type=reinterpret
      settings: infoedit="Changes signal type without altering the binary representation.   You can changed the signal between signed and unsigned, and relocate the binary point.<br><br>Hardware notes: In hardware this block costs nothing.<br><br>Example:  Suppose the input is 6 bits wide, signed, with 2 fractional bits, and the output is forced to unsigned with 0 fractional bits.  Then an input of -2.0 (1110.00 in binary 2's complement) becomes an output of 56 (111000 in binary)."
  sign0_{0..7} (8 alike) : xbsIndex_r4/Slice  nbits=1  boolean_output=off  mode=Upper Bit Location + Width  bit1=0  base1=MSB of Input  bit0=0  base0=MSB of Input  dbl_ovrd=off  block_type=slice
  slc0 : xbsIndex_r4/Slice  nbits=1  boolean_output=off  mode=Lower Bit Location + Width  bit1=0  base1=MSB of Input  bit0=0  base0=LSB of Input  dbl_ovrd=off  block_type=slice
  slc1 : xbsIndex_r4/Slice  nbits=6  boolean_output=off  mode=Lower Bit Location + Width  bit1=0  base1=MSB of Input  bit0=0  base0=LSB of Input  dbl_ovrd=off  block_type=slice
  slc2 : xbsIndex_r4/Slice  nbits=1  boolean_output=off  mode=Lower Bit Location + Width  bit1=0  base1=MSB of Input  bit0=0  base0=LSB of Input  dbl_ovrd=off  block_type=slice
  slc3 : xbsIndex_r4/Slice  nbits=6  boolean_output=off  mode=Lower Bit Location + Width  bit1=0  base1=MSB of Input  bit0=0  base0=LSB of Input  dbl_ovrd=off  block_type=slice
  slc4 : xbsIndex_r4/Slice  nbits=14  boolean_output=off  mode=Lower Bit Location + Width  bit1=0  base1=MSB of Input  bit0=0  base0=LSB of Input  dbl_ovrd=off  block_type=slice
  sync_del0 : simulink/Discrete/Integer Delay  vinit=0.0  samptime=-1  NumDelays=2
  sync_del1 : simulink/Discrete/Integer Delay  vinit=0.0  samptime=-1  NumDelays=1
  sync_del2 : simulink/Discrete/Integer Delay  vinit=0.0  samptime=-1  NumDelays=1
  sync_del3 : simulink/Discrete/Integer Delay  vinit=0.0  samptime=-1  NumDelays=1
  sync_ds0 : dspsigops/Downsample  N=8  phase=0  ic=0  smode=Allow multirate  fmode=Maintain input frame size
  sync_ds1 : dspsigops/Downsample  N=8  phase=2  ic=0  smode=Allow multirate  fmode=Maintain input frame size
  sync_ds2 : dspsigops/Downsample  N=8  phase=4  ic=0  smode=Allow multirate  fmode=Maintain input frame size
  sync_ds3 : dspsigops/Downsample  N=8  phase=6  ic=0  smode=Allow multirate  fmode=Maintain input frame size
  test_kat_adc_fab_inter_katadc1_gain_load : xbsIndex_r4/Gateway Out  hdl_port=on  timing_constraint=None  locs_specified=off  LOCs={}  block_type=gatewayout
      settings: infoedit="Gateway out block.  Converts Xilinx fixed point inputs into ouputs of type Simulink integer, double, or fixed point.<br><br>Hardware notes:  In hardware these blocks become top level output ports or are discarded, depending on how they are configured."  block_version=11.4
  test_kat_adc_fab_inter_katadc1_gain_value : xbsIndex_r4/Gateway Out  hdl_port=on  timing_constraint=None  locs_specified=off  LOCs={}  block_type=gatewayout
      settings: infoedit="Gateway out block.  Converts Xilinx fixed point inputs into ouputs of type Simulink integer, double, or fixed point.<br><br>Hardware notes:  In hardware these blocks become top level output ports or are discarded, depending on how they are configured."  block_version=11.4
  test_kat_adc_fab_inter_katadc1_user_data_valid : xbsIndex_r4/Gateway In  arith_type=Boolean  n_bits=16  bin_pt=14  quantization="Round  (unbiased: +/- Inf)"  overflow=Saturate  period=1  dbl_ovrd=off  timing_constraint=None  locs_specified=off  LOCs={}  hdl_port=on  block_type=gatewayin
      settings: infoedit="Gateway in block.  Converts inputs of type Simulink integer, double and fixed point to  Xilinx fixed point type.<br><br>Hardware notes:  In hardware these blocks become top level input ports."  block_version=11.4
  test_kat_adc_fab_inter_katadc1_user_datai{0..3} (4 alike) : xbsIndex_r4/Gateway In  arith_type="Signed  (2's comp)"  n_bits=8  bin_pt=0  quantization="Round  (unbiased: +/- Inf)"  overflow=Saturate  period=1  dbl_ovrd=off  timing_constraint=None  locs_specified=off  LOCs={}  hdl_port=on  block_type=gatewayin
      settings: infoedit="Gateway in block.  Converts inputs of type Simulink integer, double and fixed point to  Xilinx fixed point type.<br><br>Hardware notes:  In hardware these blocks become top level input ports."  block_version=11.4
  test_kat_adc_fab_inter_katadc1_user_dataq{0..3} (4 alike) : xbsIndex_r4/Gateway In  arith_type="Signed  (2's comp)"  n_bits=8  bin_pt=0  quantization="Round  (unbiased: +/- Inf)"  overflow=Saturate  period=1  dbl_ovrd=off  timing_constraint=None  locs_specified=off  LOCs={}  hdl_port=on  block_type=gatewayin
      settings: infoedit="Gateway in block.  Converts inputs of type Simulink integer, double and fixed point to  Xilinx fixed point type.<br><br>Hardware notes:  In hardware these blocks become top level input ports."  block_version=11.4
  test_kat_adc_fab_inter_katadc1_user_outofrange0 : xbsIndex_r4/Gateway In  arith_type=Boolean  n_bits=16  bin_pt=14  quantization="Round  (unbiased: +/- Inf)"  overflow=Saturate  period=1  dbl_ovrd=off  timing_constraint=None  locs_specified=off  LOCs={}  hdl_port=on  block_type=gatewayin
      settings: infoedit="Gateway in block.  Converts inputs of type Simulink integer, double and fixed point to  Xilinx fixed point type.<br><br>Hardware notes:  In hardware these blocks become top level input ports."  block_version=11.4
  test_kat_adc_fab_inter_katadc1_user_outofrange1 : xbsIndex_r4/Gateway In  arith_type=Boolean  n_bits=16  bin_pt=14  quantization="Round  (unbiased: +/- Inf)"  overflow=Saturate  period=1  dbl_ovrd=off  timing_constraint=None  locs_specified=off  LOCs={}  hdl_port=on  block_type=gatewayin
      settings: infoedit="Gateway in block.  Converts inputs of type Simulink integer, double and fixed point to  Xilinx fixed point type.<br><br>Hardware notes:  In hardware these blocks become top level input ports."  block_version=11.4
  test_kat_adc_fab_inter_katadc1_user_sync{0..3} (4 alike) : xbsIndex_r4/Gateway In  arith_type=Boolean  n_bits=16  bin_pt=14  quantization="Round  (unbiased: +/- Inf)"  overflow=Saturate  period=1  dbl_ovrd=off  timing_constraint=None  locs_specified=off  LOCs={}  hdl_port=on  block_type=gatewayin
      settings: infoedit="Gateway in block.  Converts inputs of type Simulink integer, double and fixed point to  Xilinx fixed point type.<br><br>Hardware notes:  In hardware these blocks become top level input ports."  block_version=11.4
  trigger : xbsIndex_r4/Constant  arith_type=Unsigned  const=1  n_bits=1  bin_pt=0  explicit_period=off  period=1  equ=P=C  opselect=C  inp2=PCIN>>17  opr=+  inp1=P  carry=CIN  dbl_ovrd=off  block_type=constant
      settings: block_version=11.4
  val0_{0..7} (8 alike) : xbsIndex_r4/Slice  nbits=7  boolean_output=off  mode=Lower Bit Location + Width  bit1=0  base1=LSB of Input  bit0=0  base0=LSB of Input  dbl_ovrd=off  block_type=slice
  data0_0 : Outport
  data0_1 : Outport  Port=2
  data0_2 : Outport  Port=3
  data0_3 : Outport  Port=4
  data0_4 : Outport  Port=5
  data0_5 : Outport  Port=6
  data0_6 : Outport  Port=7
  data0_7 : Outport  Port=8
  or0 : Outport  Port=9
  or1 : Outport  Port=10
  sync0 : Outport  Port=11
  sync1 : Outport  Port=12
  sync2 : Outport  Port=13
  sync3 : Outport  Port=14
  data_valid : Outport  Port=15
  wires:
  sim_data0/1 -> gain0/1
  gain0/1 -> bias0/1
  bias0/1 -> d0_ds0/1, d0_ds1/1, d0_ds2/1, d0_ds3/1, d0_ds4/1, d0_ds5/1, d0_ds6/1, d0_ds7/1
  d0_ds0/1 -> d0_del0/1
  d0_del0/1 -> test_kat_adc_fab_inter_katadc1_user_datai0/1, lt0_0/1, gt0_0/1
  test_kat_adc_fab_inter_katadc1_user_datai0/1 -> sign0_0/1, val0_0/1
  sign0_0/1 -> inv0_0/1
  inv0_0/1 -> concat0_0/1
  val0_0/1 -> concat0_0/2
  concat0_0/1 -> reinterpret0_0/1
  reinterpret0_0/1 -> data0_0/1
  d0_ds1/1 -> d0_del1/1
  d0_del1/1 -> test_kat_adc_fab_inter_katadc1_user_dataq0/1, lt0_1/1, gt0_1/1
  test_kat_adc_fab_inter_katadc1_user_dataq0/1 -> sign0_1/1, val0_1/1
  sign0_1/1 -> inv0_1/1
  inv0_1/1 -> concat0_1/1
  val0_1/1 -> concat0_1/2
  concat0_1/1 -> reinterpret0_1/1
  reinterpret0_1/1 -> data0_1/1
  d0_ds2/1 -> d0_del2/1
  d0_del2/1 -> test_kat_adc_fab_inter_katadc1_user_datai1/1, lt0_2/1, gt0_2/1
  test_kat_adc_fab_inter_katadc1_user_datai1/1 -> sign0_2/1, val0_2/1
  sign0_2/1 -> inv0_2/1
  inv0_2/1 -> concat0_2/1
  val0_2/1 -> concat0_2/2
  concat0_2/1 -> reinterpret0_2/1
  reinterpret0_2/1 -> data0_2/1
  d0_ds3/1 -> d0_del3/1
  d0_del3/1 -> test_kat_adc_fab_inter_katadc1_user_dataq1/1, lt0_3/1, gt0_3/1
  test_kat_adc_fab_inter_katadc1_user_dataq1/1 -> sign0_3/1, val0_3/1
  sign0_3/1 -> inv0_3/1
  inv0_3/1 -> concat0_3/1
  val0_3/1 -> concat0_3/2
  concat0_3/1 -> reinterpret0_3/1
  reinterpret0_3/1 -> data0_3/1
  d0_ds4/1 -> d0_del4/1
  d0_del4/1 -> test_kat_adc_fab_inter_katadc1_user_datai2/1, lt0_4/1, gt0_4/1
  test_kat_adc_fab_inter_katadc1_user_datai2/1 -> sign0_4/1, val0_4/1
  sign0_4/1 -> inv0_4/1
  inv0_4/1 -> concat0_4/1
  val0_4/1 -> concat0_4/2
  concat0_4/1 -> reinterpret0_4/1
  reinterpret0_4/1 -> data0_4/1
  d0_ds5/1 -> d0_del5/1
  d0_del5/1 -> test_kat_adc_fab_inter_katadc1_user_dataq2/1, lt0_5/1, gt0_5/1
  test_kat_adc_fab_inter_katadc1_user_dataq2/1 -> sign0_5/1, val0_5/1
  sign0_5/1 -> inv0_5/1
  inv0_5/1 -> concat0_5/1
  val0_5/1 -> concat0_5/2
  concat0_5/1 -> reinterpret0_5/1
  reinterpret0_5/1 -> data0_5/1
  d0_ds6/1 -> d0_del6/1
  d0_del6/1 -> test_kat_adc_fab_inter_katadc1_user_datai3/1, lt0_6/1, gt0_6/1
  test_kat_adc_fab_inter_katadc1_user_datai3/1 -> sign0_6/1, val0_6/1
  sign0_6/1 -> inv0_6/1
  inv0_6/1 -> concat0_6/1
  val0_6/1 -> concat0_6/2
  concat0_6/1 -> reinterpret0_6/1
  reinterpret0_6/1 -> data0_6/1
  d0_ds7/1 -> d0_del7/1
  d0_del7/1 -> test_kat_adc_fab_inter_katadc1_user_dataq3/1, lt0_7/1, gt0_7/1
  test_kat_adc_fab_inter_katadc1_user_dataq3/1 -> sign0_7/1, val0_7/1
  sign0_7/1 -> inv0_7/1
  inv0_7/1 -> concat0_7/1
  val0_7/1 -> concat0_7/2
  concat0_7/1 -> reinterpret0_7/1
  reinterpret0_7/1 -> data0_7/1
  lt0_0/1 -> logical0/1
  gt0_0/1 -> logical0/2
  lt0_1/1 -> logical0/3
  gt0_1/1 -> logical0/4
  lt0_2/1 -> logical0/5
  gt0_2/1 -> logical0/6
  lt0_3/1 -> logical0/7
  gt0_3/1 -> logical0/8
  lt0_4/1 -> logical0/9
  gt0_4/1 -> logical0/10
  lt0_5/1 -> logical0/11
  gt0_5/1 -> logical0/12
  lt0_6/1 -> logical0/13
  gt0_6/1 -> logical0/14
  lt0_7/1 -> logical0/15
  gt0_7/1 -> logical0/16
  logical0/1 -> test_kat_adc_fab_inter_katadc1_user_outofrange0/1, test_kat_adc_fab_inter_katadc1_user_outofrange1/1
  test_kat_adc_fab_inter_katadc1_user_outofrange0/1 -> or0/1
  test_kat_adc_fab_inter_katadc1_user_outofrange1/1 -> or1/1
  sim_sync/1 -> sync_ds0/1, sync_ds1/1, sync_ds2/1, sync_ds3/1
  sync_ds0/1 -> sync_del0/1
  sync_del0/1 -> test_kat_adc_fab_inter_katadc1_user_sync0/1
  test_kat_adc_fab_inter_katadc1_user_sync0/1 -> sync0/1
  sync_ds1/1 -> sync_del1/1
  sync_del1/1 -> test_kat_adc_fab_inter_katadc1_user_sync1/1
  test_kat_adc_fab_inter_katadc1_user_sync1/1 -> sync1/1
  sync_ds2/1 -> sync_del2/1
  sync_del2/1 -> test_kat_adc_fab_inter_katadc1_user_sync2/1
  test_kat_adc_fab_inter_katadc1_user_sync2/1 -> sync2/1
  sync_ds3/1 -> sync_del3/1
  sync_del3/1 -> test_kat_adc_fab_inter_katadc1_user_sync3/1
  test_kat_adc_fab_inter_katadc1_user_sync3/1 -> sync3/1
  sim_data_valid/1 -> test_kat_adc_fab_inter_katadc1_user_data_valid/1
  test_kat_adc_fab_inter_katadc1_user_data_valid/1 -> data_valid/1
  en0/1 -> slc0/1, slc2/1
  atten0/1 -> slc1/1, slc3/1
  slc1/1 -> inv0/1
  slc3/1 -> inv1/1
  trigger/1 -> con/1
  slc0/1 -> con/4
  inv0/1 -> con/5
  slc2/1 -> con/2
  inv1/1 -> con/3
  con/1 -> reg/1, changed/2
  reg/1 -> changed/1, slc4/1
  slc4/1 -> cast0/1
  cast0/1 -> test_kat_adc_fab_inter_katadc1_gain_value/1
  changed/1 -> cast1/1
  cast1/1 -> test_kat_adc_fab_inter_katadc1_gain_load/1
